simulink model "example5_hybridpid"  (R2021b)
settings: Solver=VariableStepAuto  StartTime=0.0  StopTime=10  RelTol=1e-3
settings Model: Creator=junmoon  LastModifiedBy=user

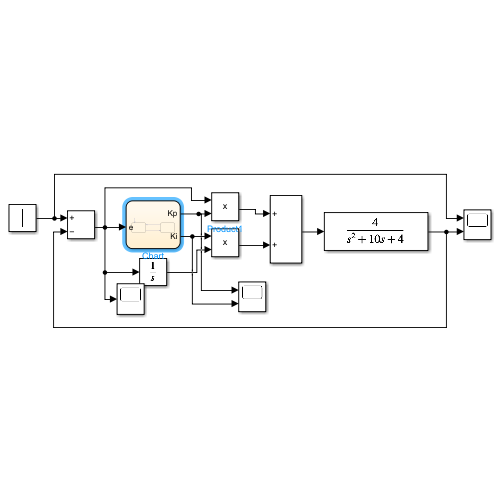
[thumbnail: Simulink's stored preview of the top-level diagram]
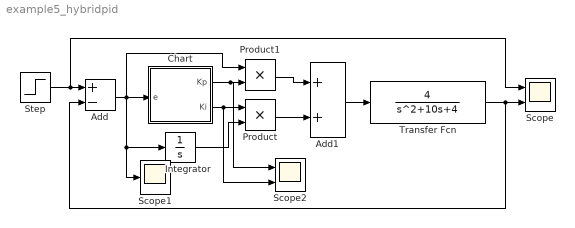
== system example5_hybridpid ==
  Add : Sum  Inputs=+-
  Add1 : Sum
  Chart : Stateflow chart  TreatAsAtomicUnit=on
  Integrator : Integrator
  Product : Product
  Product1 : Product
  Scope : Scope  NumInputPorts=2
  Scope1 : Scope
  Scope2 : Scope  NumInputPorts=2
  Step : Step  SampleTime=0.001
  Transfer Fcn : TransferFcn  Numerator=[4]  Denominator=[1 10 4]
  wires:
  Transfer Fcn/1 -> Scope/2, Add/2
  Step/1 -> Add/1, Scope/1
  Add/1 -> Product1/1, Chart/1(e), Integrator/1, Scope1/1
  Chart/1(Kp) -> Scope2/1, Product1/2
  Chart/2(Ki) -> Scope2/2, Product/1
  Product/1 -> Add1/2
  Integrator/1 -> Product/2
  Add1/1 -> Transfer Fcn/1
  Product1/1 -> Add1/1

== stateflow chart example5_hybridpid/Chart ==
  state PID1
    Kp=0.5
    Ki=0.9
  state PID2
    Kp=1
    Ki=2
  (default) -> PID1
  PID2 -> PID1 : [abs(e) <=0.1]
  PID1 -> PID2 : [abs(e) >0.1]
  data: e input; Kp output; Ki output
